simulink model "PID"  (R2018a)
settings: Solver=VariableStepAuto  StartTime=0.0  StopTime=20  RelTol=1e-3
libraries: simulink x1
settings Model: Creator=Neo  LastModifiedBy=Neo

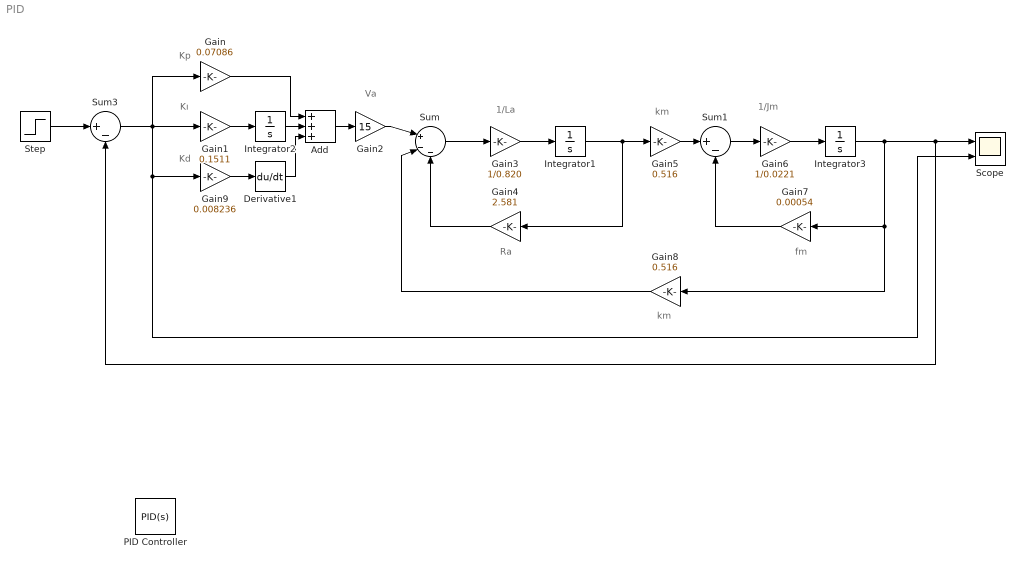
== system PID ==
  note: km
  note: Ra
  note: fm
  note: 1/Jm
  note: km
  note: 1/La
  note: Va
  note: Kd
  note: Kı
  note: Kp
  Add : Sum  Inputs=+++
  Derivative1 : Derivative
  Gain : Gain  Gain=0.07086
  Gain1 : Gain  Gain=0.1511
  Gain2 : Gain  Gain=15
  Gain3 : Gain  Gain=1/0.820
  Gain4 : Gain  Gain=2.581
  Gain5 : Gain  Gain=0.516
  Gain6 : Gain  Gain=1/0.0221
  Gain7 : Gain  Gain=0.00054
  Gain8 : Gain  Gain=0.516
  Gain9 : Gain  Gain=0.008236
  Integrator1 : Integrator
  Integrator2 : Integrator
  Integrator3 : Integrator
  PID Controller : simulink/Continuous/PID Controller  Controller=PID  TimeDomain=Continuous-time  SampleTime=-1  IntegratorMethod=Forward Euler  FilterMethod=Forward Euler  Form=Parallel  UseFilter=on  ControllerParametersSource=internal  P=0.07086  I=0.1511  D=0.008236  N=728.7  InitialConditionSource=internal  InitialConditionForIntegrator=0  InitialConditionForFilter=0  ExternalReset=none  LimitOutput=off  UpperSaturationLimit=inf  LowerSaturationLimit=-inf  LinearizeAsGain=on  AntiWindupMode=none  Kb=1  TrackingMode=off  Kt=1  PParamMin=[]  PParamMax=[]  IParamMin=[]  IParamMax=[]  DParamMin=[]  DParamMax=[]  NParamMin=[]  NParamMax=[]  KbParamMin=[]  KbParamMax=[]  KtParamMin=[]  KtParamMax=[]  POutMin=[]  POutMax=[]  IOutMin=[]  IOutMax=[]  DOutMin=[]  DOutMax=[]  NOutMin=[]  NOutMax=[]  KbOutMin=[]  KbOutMax=[]  KtOutMin=[]  KtOutMax=[]  IntegratorOutMin=[]  IntegratorOutMax=[]  FilterOutMin=[]  FilterOutMax=[]  SumOutMin=[]  SumOutMax=[]  SumI1OutMin=[]  SumI1OutMax=[]  SumI2OutMin=[]  SumI2OutMax=[]  SumI3OutMin=[]  SumI3OutMax=[]  SumDOutMin=[]  SumDOutMax=[]  SaturationOutMin=[]  SaturationOutMax=[]  IntegratorContinuousStateAttributes=''  IntegratorStateMustResolveToSignalObject=off  IntegratorRTWStateStorageClass=Auto  FilterContinuousStateAttributes=''  FilterStateMustResolveToSignalObject=off  FilterRTWStateStorageClass=Auto  DifferentiatorICPrevScaledInput=0  DifferentiatorOutMin=[]  DifferentiatorOutMax=[]  FilterDiffOutCoefMin=[]  FilterDiffOutCoefMax=[]  SumDenOutMin=[]  SumDenOutMax=[]  SumNumOutMin=[]  SumNumOutMax=[]  ReciprocalOutMin=[]  ReciprocalOutMax=[]  DivideOutMin=[]  DivideOutMax=[]  TunerSelectOption=Transfer Function Based (PID Tuner App)
  Scope : Scope  NumInputPorts=2
  Step : Step  Time=0  Before=1  After=100  SampleTime=0
  Sum : Sum  Inputs=|+--
  Sum1 : Sum  Inputs=|+-
  Sum3 : Sum  Inputs=|+-
  wires:
  Gain1/1 -> Integrator2/1
  Gain9/1 -> Derivative1/1
  Gain2/1 -> Sum/1
  Sum/1 -> Gain3/1
  Gain3/1 -> Integrator1/1
  Integrator1/1 -> Gain5/1, Gain4/1
  Gain6/1 -> Integrator3/1
  Gain5/1 -> Sum1/1
  Sum1/1 -> Gain6/1
  Gain7/1 -> Sum1/2
  Gain4/1 -> Sum/3
  Gain8/1 -> Sum/2
  Integrator3/1 -> Scope/1, Sum3/2, Gain8/1, Gain7/1
  Sum3/1 -> Gain/1, Gain9/1, Scope/2, Gain1/1
  Step/1 -> Sum3/1
  Integrator2/1 -> Add/2
  Add/1 -> Gain2/1
  Gain/1 -> Add/1
  Derivative1/1 -> Add/3
